simulink model "Heat_Exchanger"  (R2024a)
settings: Solver=FixedStepAuto  StartTime=0.0  StopTime=Inf  RelTol=1e-3
model workspace (MAT data in the model file):
  Avg_HI = 400
  PLC_IP_Address = '127.0.0.1'
libraries: dspnetwork x26
settings Model: Creator=antho  LastModifiedBy=chach
settings SolverCC: AlgebraicLoopSolver=TrustRegion
settings DataIOCC: ReturnWorkspaceOutputs=off
settings OptimizationCC: LifeSpan=inf
settings DebuggingCC: UnconnectedInputMsg=warning  UnconnectedOutputMsg=warning  UnconnectedLineMsg=warning  SFExecutionAtInitializationDiag=none  ArithmeticOperatorsInVariantConditions=warning
settings ModelReferenceCC: EnableRefExpFcnMdlSchedulingChecks=on
settings SFSimCC: SimUseLocalCustomCode=off  CustomCodeUndefinedFunction=UseInterfaceOnly
settings RTWCC: PackageGeneratedCodeAndArtifacts=on  PackageName=Heat_Exchanger  RTWUseLocalCustomCode=off  GPUComputeCapability=3.5
settings CodeAppCC: StateflowObjectComments=on

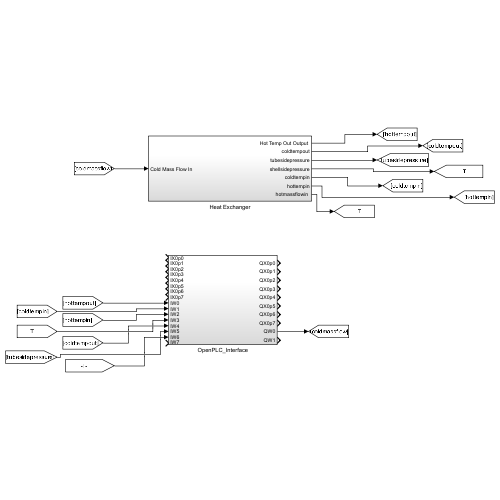
[thumbnail: Simulink's stored preview of the top-level diagram]
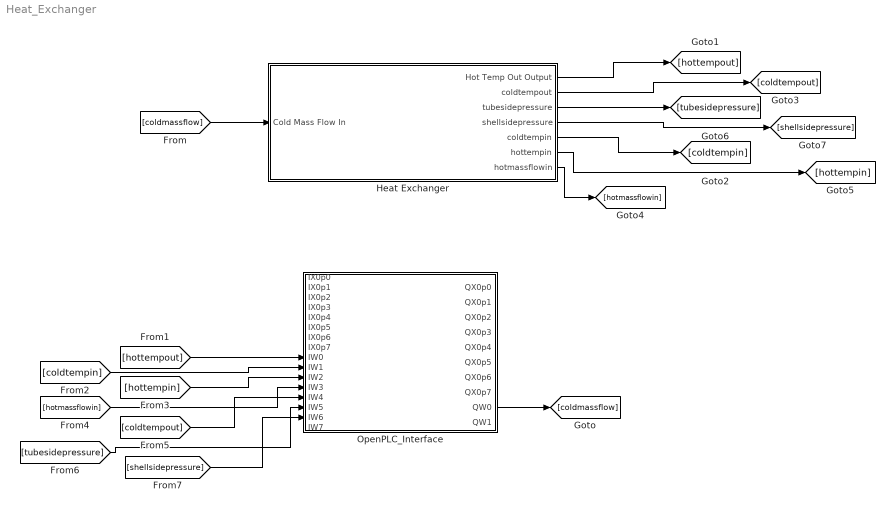
== system Heat_Exchanger ==
  Heat Exchanger : Subsystem
  OpenPLC_Interface : Subsystem
  wires:
  OpenPLC_Interface/9(QW0) -> [coldmassflow]
  [hottempout] -> OpenPLC_Interface/9(IW0)
  [coldtempin] -> OpenPLC_Interface/10(IW1)
  [hottempin] -> OpenPLC_Interface/11(IW2)
  [hotmassflowin] -> OpenPLC_Interface/12(IW3)
  [coldtempout] -> OpenPLC_Interface/13(IW4)
  [tubesidepressure] -> OpenPLC_Interface/14(IW5)
  [shellsidepressure] -> OpenPLC_Interface/15(IW6)
  Heat Exchanger/1("Hot Temp Out Output ") -> [hottempout]
  Heat Exchanger/2(coldtempout) -> [coldtempout]
  Heat Exchanger/3(tubesidepressure) -> [tubesidepressure]
  Heat Exchanger/4(shellsidepressure) -> [shellsidepressure]
  Heat Exchanger/5(coldtempin) -> [coldtempin]
  Heat Exchanger/7("hotmassflowin ") -> [hotmassflowin]
  Heat Exchanger/6(hottempin) -> [hottempin]
  [coldmassflow] -> Heat Exchanger/1(Cold Mass Flow In)

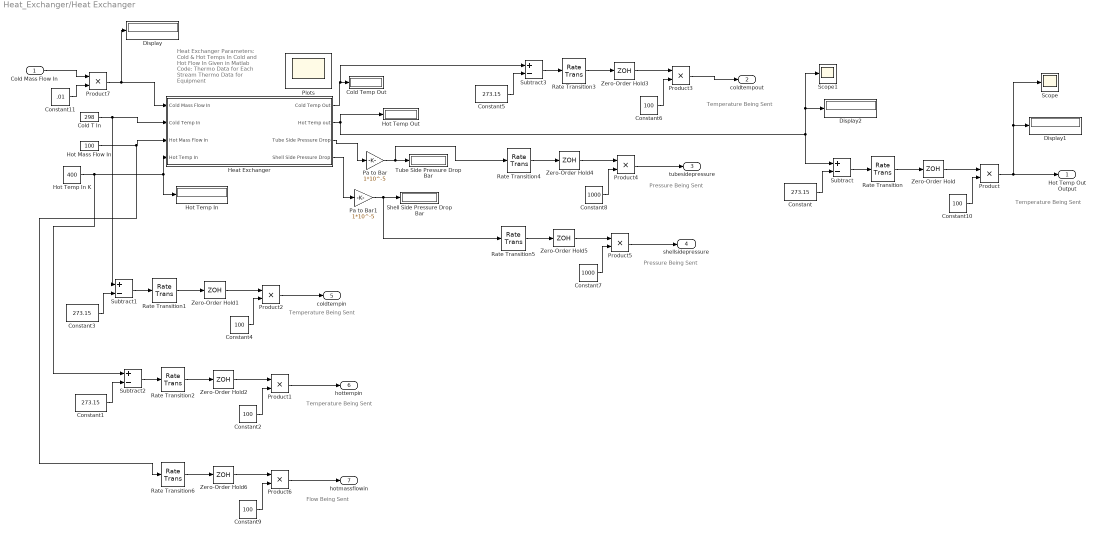
== system Heat_Exchanger/Heat Exchanger ==
  note: Heat Exchanger Parameters:
      | Cold & Hot Temps In
      | Cold and Hot Flow In
      | Given in Matlab Code:
      | Thermo Data for Each Stream
      | Thermo Data for Equipment
  note: Temperature Being Sent
  note: Temperature Being Sent
  note: Temperature Being Sent
  note: Pressure Being Sent
  note: Pressure Being Sent
  note: Flow Being Sent
  note: Temperature Being Sent
  Cold Mass Flow In : Inport
  Cold T In : Constant  Value=298
  Cold Temp Out : Display
  Constant{,1,3,5} (4 alike) : Constant  Value=273.15
  Constant{2,4,6,9..10} (5 alike) : Constant  Value=100
  Constant11 : Constant  Value=.01
  Constant7 : Constant  Value=1000
  Constant8 : Constant  Value=1000
  Display : Display
  Display1 : Display
  Display2 : Display
  Heat Exchanger : Subsystem
  Hot Mass Flow In : Constant  Value=100
  Hot Temp In : Display
  Hot Temp In K : Constant  Value=400
  Hot Temp Out : Display
  Pa to Bar : Gain  Gain=1*10^-5
  Pa to Bar1 : Gain  Gain=1*10^-5
  Plots : Scope
      settings: Floating=on
  Product{,1..7} (8 alike) : Product
  Rate Transition{,1..6} (7 alike) : RateTransition
  Scope : Scope
  Scope1 : Scope
  Shell Side Pressure Drop Bar : Display
  Subtract{,1..3} (4 alike) : Sum  Inputs=+-
  Tube Side Pressure Drop Bar : Display
  Zero-Order Hold{,1..6} (7 alike) : ZeroOrderHold  SampleTime=0.1
  "Hot Temp Out Output " : Outport
  coldtempout : Outport  Port=2
  tubesidepressure : Outport  Port=3
  shellsidepressure : Outport  Port=4
  coldtempin : Outport  Port=5
  hottempin : Outport  Port=6
  "hotmassflowin " : Outport  Port=7
  wires:
  Heat Exchanger/1(Cold Temp Out) -> Subtract3/1, Cold Temp Out/1
  Cold T In/1 -> Subtract1/1, Heat Exchanger/2(Cold Temp In)
  Hot Temp In K/1 -> Subtract2/1, Heat Exchanger/4(Hot Temp In), Hot Temp In/1
  Hot Mass Flow In/1 -> Rate Transition6/1, Heat Exchanger/3(Hot Mass Flow In)
  Pa to Bar/1 -> Rate Transition4/1, Tube Side Pressure Drop Bar/1
  Heat Exchanger/3(Tube Side Pressure Drop) -> Pa to Bar/1
  Pa to Bar1/1 -> Rate Transition5/1, Shell Side Pressure Drop Bar/1
  Heat Exchanger/4(Shell Side Pressure Drop) -> Pa to Bar1/1
  Product2/1 -> coldtempin/1
  Subtract1/1 -> Rate Transition1/1
  Zero-Order Hold1/1 -> Product2/1
  Constant4/1 -> Product2/2
  Constant3/1 -> Subtract1/2
  Rate Transition1/1 -> Zero-Order Hold1/1
  Product1/1 -> hottempin/1
  Subtract2/1 -> Rate Transition2/1
  Zero-Order Hold2/1 -> Product1/1
  Constant2/1 -> Product1/2
  Constant1/1 -> Subtract2/2
  Rate Transition2/1 -> Zero-Order Hold2/1
  Product3/1 -> coldtempout/1
  Subtract3/1 -> Rate Transition3/1
  Zero-Order Hold3/1 -> Product3/1
  Constant6/1 -> Product3/2
  Constant5/1 -> Subtract3/2
  Rate Transition3/1 -> Zero-Order Hold3/1
  Product4/1 -> tubesidepressure/1
  Zero-Order Hold4/1 -> Product4/1
  Constant8/1 -> Product4/2
  Rate Transition4/1 -> Zero-Order Hold4/1
  Zero-Order Hold5/1 -> Product5/1
  Product5/1 -> shellsidepressure/1
  Rate Transition5/1 -> Zero-Order Hold5/1
  Constant7/1 -> Product5/2
  Zero-Order Hold6/1 -> Product6/1
  Product6/1 -> "hotmassflowin "/1
  Rate Transition6/1 -> Zero-Order Hold6/1
  Constant9/1 -> Product6/2
  Subtract/1 -> Rate Transition/1
  Heat Exchanger/2(Hot Temp out) -> Subtract/1, Scope1/1, Display2/1, Hot Temp Out/1
  Constant10/1 -> Product/2
  Constant/1 -> Subtract/2
  Rate Transition/1 -> Zero-Order Hold/1
  Product/1 -> "Hot Temp Out Output "/1, Scope/1, Display1/1
  Zero-Order Hold/1 -> Product/1
  Constant11/1 -> Product7/2
  Cold Mass Flow In/1 -> Product7/1
  Product7/1 -> Display/1, Heat Exchanger/1(Cold Mass Flow In)

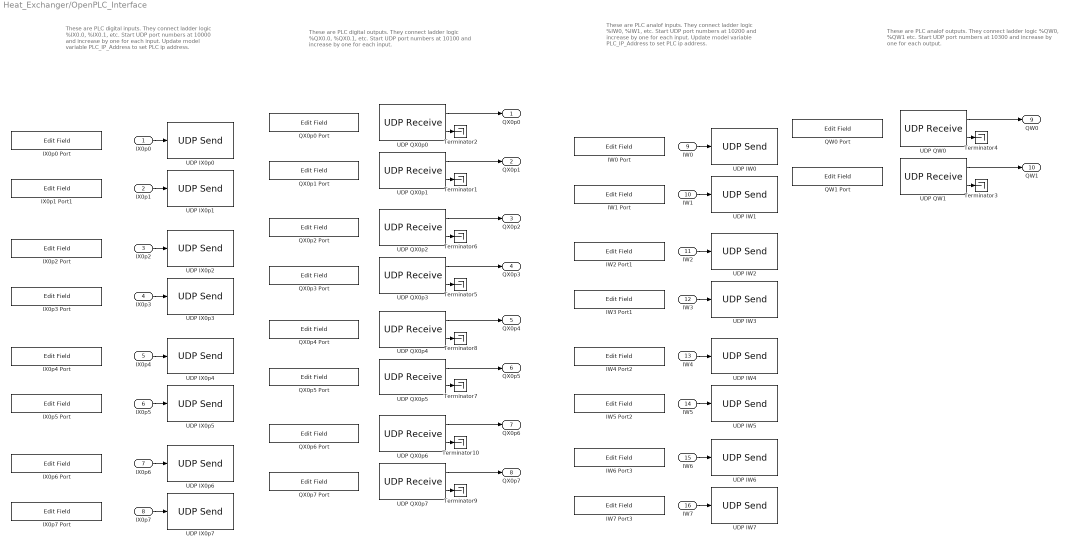
== system Heat_Exchanger/OpenPLC_Interface ==
  note: These are PLC digital inputs. They connect
      | ladder logic %IX0.0, %IX0.1, etc.
      |
      | Start UDP port numbers at 10000 and
      | increase by one for each input.
      |
      | Update model variable PLC_IP_Address
      | to set PLC ip address.
  note: These are PLC digital outputs. They connect
      | ladder logic %QX0.0, %QX0.1, etc.
      |
      | Start UDP port numbers at 10100 and increase
      | by one for each input.
  note: These are PLC analof inputs. They connect
      | ladder logic %IW0, %IW1, etc.
      |
      | Start UDP port numbers  at 10200 and
      | increase by one for each input.
      |
      | Update model variable PLC_IP_Address
      | to set PLC ip address.
  note: These are PLC analof outputs. They connect
      | ladder logic %QW0, %QW1 etc.
      |
      | Start UDP port numbers at 10300 and increase
      | by one for each output.
  "IX0p0 " : Inport
  IX0p1 : Inport  Port=2
  IX0p2 : Inport  Port=3
  IX0p3 : Inport  Port=4
  IX0p4 : Inport  Port=5
  IX0p5 : Inport  Port=6
  IX0p6 : Inport  Port=7
  IX0p7 : Inport  Port=8
  IW0 : Inport  Port=9
  IW1 : Inport  Port=10
  IW2 : Inport  Port=11
  IW3 : Inport  Port=12
  IW4 : Inport  Port=13
  IW5 : Inport  Port=14
  IW6 : Inport  Port=15
  IW7 : Inport  Port=16
  IW0 Port : EditField  LabelPosition=Hide  ShowInitialText=on  Alignment=Center
  IW1 Port : EditField  LabelPosition=Hide  ShowInitialText=on  Alignment=Center
  IW2 Port1 : EditField  LabelPosition=Hide  ShowInitialText=on  Alignment=Center
  IW3 Port1 : EditField  LabelPosition=Hide  ShowInitialText=on  Alignment=Center
  IW4 Port2 : EditField  LabelPosition=Hide  ShowInitialText=on  Alignment=Center
  IW5 Port2 : EditField  LabelPosition=Hide  ShowInitialText=on  Alignment=Center
  IW6 Port3 : EditField  LabelPosition=Hide  ShowInitialText=on  Alignment=Center
  IW7 Port3 : EditField  LabelPosition=Hide  ShowInitialText=on  Alignment=Center
  IX0p0 Port : EditField  LabelPosition=Hide  ShowInitialText=on  Alignment=Center
  IX0p1 Port1 : EditField  LabelPosition=Hide  ShowInitialText=on  Alignment=Center
  IX0p2 Port : EditField  LabelPosition=Hide  ShowInitialText=on  Alignment=Center
  IX0p3 Port : EditField  LabelPosition=Hide  ShowInitialText=on  Alignment=Center
  IX0p4 Port : EditField  LabelPosition=Hide  ShowInitialText=on  Alignment=Center
  IX0p5 Port : EditField  LabelPosition=Hide  ShowInitialText=on  Alignment=Center
  IX0p6 Port : EditField  LabelPosition=Hide  ShowInitialText=on  Alignment=Center
  IX0p7 Port : EditField  LabelPosition=Hide  ShowInitialText=on  Alignment=Center
  QW0 Port : EditField  LabelPosition=Hide  ShowInitialText=on  Alignment=Center
  QW1 Port : EditField  LabelPosition=Hide  ShowInitialText=on  Alignment=Center
  QX0p0 Port : EditField  LabelPosition=Hide  ShowInitialText=on  Alignment=Center
  QX0p1 Port : EditField  LabelPosition=Hide  ShowInitialText=on  Alignment=Center
  QX0p2 Port : EditField  LabelPosition=Hide  ShowInitialText=on  Alignment=Center
  QX0p3 Port : EditField  LabelPosition=Hide  ShowInitialText=on  Alignment=Center
  QX0p4 Port : EditField  LabelPosition=Hide  ShowInitialText=on  Alignment=Center
  QX0p5 Port : EditField  LabelPosition=Hide  ShowInitialText=on  Alignment=Center
  QX0p6 Port : EditField  LabelPosition=Hide  ShowInitialText=on  Alignment=Center
  QX0p7 Port : EditField  LabelPosition=Hide  ShowInitialText=on  Alignment=Center
  Terminator{1..10} (10 alike) : Terminator
  UDP IW0 : dspnetwork/UDP Send  remoteURL='localhost'  remotePort=10200  localURL='255.255.255.255'  localPortSource=Automatically determine  localPort=-1  sendBufferSize=8192  sampletime=-1  blockPlatform=LINUX  separateLengthPort=0
  UDP IW1 : dspnetwork/UDP Send  remoteURL='localhost'  remotePort=10201  localURL='255.255.255.255'  localPortSource=Automatically determine  localPort=-1  sendBufferSize=8192  sampletime=-1  blockPlatform=LINUX  separateLengthPort=0
  UDP IW2 : dspnetwork/UDP Send  remoteURL='localhost'  remotePort=10202  localURL='255.255.255.255'  localPortSource=Automatically determine  localPort=-1  sendBufferSize=8192  sampletime=-1  blockPlatform=LINUX  separateLengthPort=0
  UDP IW3 : dspnetwork/UDP Send  remoteURL='localhost'  remotePort=10203  localURL='255.255.255.255'  localPortSource=Automatically determine  localPort=-1  sendBufferSize=8192  sampletime=-1  blockPlatform=LINUX  separateLengthPort=0
  UDP IW4 : dspnetwork/UDP Send  remoteURL='localhost'  remotePort=10204  localURL='255.255.255.255'  localPortSource=Automatically determine  localPort=-1  sendBufferSize=8192  sampletime=-1  blockPlatform=LINUX  separateLengthPort=0
  UDP IW5 : dspnetwork/UDP Send  remoteURL='localhost'  remotePort=10205  localURL='255.255.255.255'  localPortSource=Automatically determine  localPort=-1  sendBufferSize=8192  sampletime=-1  blockPlatform=LINUX  separateLengthPort=0
  UDP IW6 : dspnetwork/UDP Send  remoteURL='localhost'  remotePort=10206  localURL='255.255.255.255'  localPortSource=Automatically determine  localPort=-1  sendBufferSize=8192  sampletime=-1  blockPlatform=LINUX  separateLengthPort=0
  UDP IW7 : dspnetwork/UDP Send  remoteURL='localhost'  remotePort=10207  localURL='255.255.255.255'  localPortSource=Automatically determine  localPort=-1  sendBufferSize=8192  sampletime=-1  blockPlatform=LINUX  separateLengthPort=0
  UDP IX0p0 : dspnetwork/UDP Send  remoteURL='localhost'  remotePort=10000  localURL='255.255.255.255'  localPortSource=Automatically determine  localPort=-1  sendBufferSize=8192  sampletime=-1  blockPlatform=LINUX  separateLengthPort=0
  UDP IX0p1 : dspnetwork/UDP Send  remoteURL='localhost'  remotePort=10001  localURL='255.255.255.255'  localPortSource=Automatically determine  localPort=-1  sendBufferSize=8192  sampletime=-1  blockPlatform=LINUX  separateLengthPort=0
  UDP IX0p2 : dspnetwork/UDP Send  remoteURL='localhost'  remotePort=10002  localURL='255.255.255.255'  localPortSource=Automatically determine  localPort=-1  sendBufferSize=8192  sampletime=-1  blockPlatform=LINUX  separateLengthPort=0
  UDP IX0p3 : dspnetwork/UDP Send  remoteURL='localhost'  remotePort=10003  localURL='255.255.255.255'  localPortSource=Automatically determine  localPort=-1  sendBufferSize=8192  sampletime=-1  blockPlatform=LINUX  separateLengthPort=0
  UDP IX0p4 : dspnetwork/UDP Send  remoteURL='localhost'  remotePort=10004  localURL='255.255.255.255'  localPortSource=Automatically determine  localPort=-1  sendBufferSize=8192  sampletime=-1  blockPlatform=LINUX  separateLengthPort=0
  UDP IX0p5 : dspnetwork/UDP Send  remoteURL='localhost'  remotePort=10005  localURL='255.255.255.255'  localPortSource=Automatically determine  localPort=-1  sendBufferSize=8192  sampletime=-1  blockPlatform=LINUX  separateLengthPort=0
  UDP IX0p6 : dspnetwork/UDP Send  remoteURL='localhost'  remotePort=10006  localURL='255.255.255.255'  localPortSource=Automatically determine  localPort=-1  sendBufferSize=8192  sampletime=-1  blockPlatform=LINUX  separateLengthPort=0
  UDP IX0p7 : dspnetwork/UDP Send  remoteURL='localhost'  remotePort=10007  localURL='255.255.255.255'  localPortSource=Automatically determine  localPort=-1  sendBufferSize=8192  sampletime=-1  blockPlatform=LINUX  separateLengthPort=0
  UDP QW0 : dspnetwork/UDP Receive  localURL='0.0.0.0'  localPort=10300  remoteURL='0.0.0.0'  remotePort=-1  recvBufferSize=2  dims=1  signalDatatype=uint16  isComplex=off  isVarSize=off  showBlockingTime=on  blockingTime=0  sampletime=0.01  blockPlatform=LINUX
  UDP QW1 : dspnetwork/UDP Receive  localURL='0.0.0.0'  localPort=10301  remoteURL='0.0.0.0'  remotePort=-1  recvBufferSize=2  dims=1  signalDatatype=uint16  isComplex=off  isVarSize=off  showBlockingTime=on  blockingTime=0  sampletime=0.01  blockPlatform=LINUX
  UDP QX0p0 : dspnetwork/UDP Receive  localURL='0.0.0.0'  localPort=10100  remoteURL='0.0.0.0'  remotePort=-1  recvBufferSize=2  dims=1  signalDatatype=uint16  isComplex=off  isVarSize=off  showBlockingTime=on  blockingTime=0  sampletime=0.01  blockPlatform=LINUX
  UDP QX0p1 : dspnetwork/UDP Receive  localURL='0.0.0.0'  localPort=10101  remoteURL='0.0.0.0'  remotePort=-1  recvBufferSize=2  dims=1  signalDatatype=uint16  isComplex=off  isVarSize=off  showBlockingTime=on  blockingTime=0  sampletime=0.01  blockPlatform=LINUX
  UDP QX0p2 : dspnetwork/UDP Receive  localURL='0.0.0.0'  localPort=10102  remoteURL='0.0.0.0'  remotePort=-1  recvBufferSize=2  dims=1  signalDatatype=uint16  isComplex=off  isVarSize=off  showBlockingTime=on  blockingTime=0  sampletime=0.01  blockPlatform=LINUX
  UDP QX0p3 : dspnetwork/UDP Receive  localURL='0.0.0.0'  localPort=10103  remoteURL='0.0.0.0'  remotePort=-1  recvBufferSize=2  dims=1  signalDatatype=uint16  isComplex=off  isVarSize=off  showBlockingTime=on  blockingTime=0  sampletime=0.01  blockPlatform=LINUX
  UDP QX0p4 : dspnetwork/UDP Receive  localURL='0.0.0.0'  localPort=10104  remoteURL='0.0.0.0'  remotePort=-1  recvBufferSize=2  dims=1  signalDatatype=uint16  isComplex=off  isVarSize=off  showBlockingTime=on  blockingTime=0  sampletime=0.01  blockPlatform=LINUX
  UDP QX0p5 : dspnetwork/UDP Receive  localURL='0.0.0.0'  localPort=10105  remoteURL='0.0.0.0'  remotePort=-1  recvBufferSize=2  dims=1  signalDatatype=uint16  isComplex=off  isVarSize=off  showBlockingTime=on  blockingTime=0  sampletime=0.01  blockPlatform=LINUX
  UDP QX0p6 : dspnetwork/UDP Receive  localURL='0.0.0.0'  localPort=10106  remoteURL='0.0.0.0'  remotePort=-1  recvBufferSize=2  dims=1  signalDatatype=uint16  isComplex=off  isVarSize=off  showBlockingTime=on  blockingTime=0  sampletime=0.01  blockPlatform=LINUX
  UDP QX0p7 : dspnetwork/UDP Receive  localURL='0.0.0.0'  localPort=10107  remoteURL='0.0.0.0'  remotePort=-1  recvBufferSize=2  dims=1  signalDatatype=uint16  isComplex=off  isVarSize=off  showBlockingTime=on  blockingTime=0  sampletime=0.01  blockPlatform=LINUX
  QX0p0 : Outport
  QX0p1 : Outport  Port=2
  QX0p2 : Outport  Port=3
  QX0p3 : Outport  Port=4
  QX0p4 : Outport  Port=5
  QX0p5 : Outport  Port=6
  QX0p6 : Outport  Port=7
  QX0p7 : Outport  Port=8
  QW0 : Outport  Port=9
  QW1 : Outport  Port=10
  wires:
  IX0p1/1 -> UDP IX0p1/1
  "IX0p0 "/1 -> UDP IX0p0/1
  UDP QX0p0/1 -> QX0p0/1
  UDP QX0p0/2 -> Terminator2/1
  UDP QX0p1/2 -> Terminator1/1
  UDP QX0p1/1 -> QX0p1/1
  IW1/1 -> UDP IW1/1
  IW0/1 -> UDP IW0/1
  UDP QW1/1 -> QW1/1
  UDP QW1/2 -> Terminator3/1
  UDP QW0/2 -> Terminator4/1
  UDP QW0/1 -> QW0/1
  IX0p2/1 -> UDP IX0p2/1
  IX0p3/1 -> UDP IX0p3/1
  IX0p7/1 -> UDP IX0p7/1
  IX0p6/1 -> UDP IX0p6/1
  IX0p4/1 -> UDP IX0p4/1
  IX0p5/1 -> UDP IX0p5/1
  UDP QX0p2/1 -> QX0p2/1
  UDP QX0p2/2 -> Terminator6/1
  UDP QX0p3/1 -> QX0p3/1
  UDP QX0p3/2 -> Terminator5/1
  UDP QX0p7/2 -> Terminator9/1
  UDP QX0p7/1 -> QX0p7/1
  UDP QX0p6/1 -> QX0p6/1
  UDP QX0p6/2 -> Terminator10/1
  UDP QX0p4/1 -> QX0p4/1
  UDP QX0p4/2 -> Terminator8/1
  UDP QX0p5/1 -> QX0p5/1
  UDP QX0p5/2 -> Terminator7/1
  IW3/1 -> UDP IW3/1
  IW2/1 -> UDP IW2/1
  IW5/1 -> UDP IW5/1
  IW4/1 -> UDP IW4/1
  IW7/1 -> UDP IW7/1
  IW6/1 -> UDP IW6/1

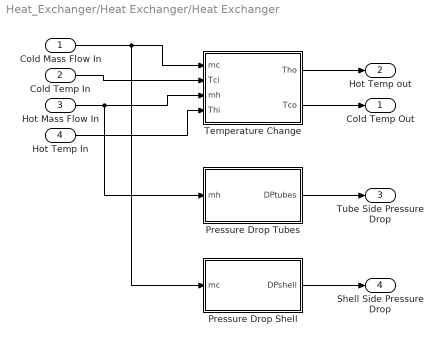
== system Heat_Exchanger/Heat Exchanger/Heat Exchanger ==
  Cold Mass Flow In : Inport
  Cold Temp In : Inport  Port=2
  Hot Mass Flow In : Inport  Port=3
  Hot Temp In : Inport  Port=4
  Pressure Drop Shell : MATLAB Function  TreatAsAtomicUnit=on
  Pressure Drop Tubes : MATLAB Function  TreatAsAtomicUnit=on
  Temperature Change : MATLAB Function  TreatAsAtomicUnit=on
  Cold Temp Out : Outport
  Hot Temp out : Outport  Port=2
  Tube Side Pressure Drop : Outport  Port=3
  Shell Side Pressure Drop : Outport  Port=4
  wires:
  Cold Temp In/1 -> Temperature Change/2(Tci)
  Hot Mass Flow In/1 -> Pressure Drop Tubes/1(mh), Temperature Change/3(mh)
  Cold Mass Flow In/1 -> Pressure Drop Shell/1(mc), Temperature Change/1(mc)
  Temperature Change/2(Tco) -> Cold Temp Out/1
  Pressure Drop Shell/1(DPshell) -> Shell Side Pressure Drop/1
  Temperature Change/1(Tho) -> Hot Temp out/1
  Pressure Drop Tubes/1(DPtubes) -> Tube Side Pressure Drop/1
  Hot Temp In/1 -> Temperature Change/4(Thi)

== matlab function Heat_Exchanger/Heat Exchanger/Heat Exchanger/Pressure Drop Tubes ==
  data: mh input; DPtubes output
function DPtubes = fcn(mh)

densityh=719.15;%kg/m^3
f=0.05;
L=10.9728; %meters
twall=0.0021082;%m
Do=0.028575;%m
Di=(Do-2*twall);
v=((mh/densityh)/24)/(3.14159*(Do-2*twall)^2/4); %Average velocity
DPtubes=f*densityh*v*L/(2*Di);

DPtubes;
end

== matlab function Heat_Exchanger/Heat Exchanger/Heat Exchanger/Temperature Change ==
  data: mc input; Tci input; mh input; Tho output; Thi input; Tco output
function [Tho, Tco]= fcn(mc,Tci,mh,Thi)
    %{
    function Tho = solve(Thi, Tci, Cph, Cpc, mh, mc, A, U) %Generates the output temp of hot stream
       Tho=0;
       n=10*(Thi-Tci)-1;
       for i=0:0.1:n %Iteratively solve for Temperature
           T=Thi-.1*i;
           %Equation to solve for Thi given a "Try Value"
           Tco=((mh*Cph)/(mc*Cpc))*(Thi-T)+Tci;
           DTlm=((T-Tci)-(Thi-Tco))/(log((T-Tci)/(Thi-Tco)));
           Thotry=Thi-((U*A)/(mh*Cph))*DTlm;
           ab=abs(Thotry-T);
           %Checks for solution to problem every iteration
           if 1>ab
               Tho=Thotry;
               break;
           end
       end
        Tho;
    end
    %%%%%%%%%%%%%%%%%%%%%%%%%%%%%%%%%%%%%%%%%%%%%%%%%%%%%%%%%%%%%%%%%%%%%%%%%%%
    function h = calch(v, mu, D, k, density, Cp, ndit)%Generates h given flow rate and heat exchanger parameters
        Re=density*v*D/mu; %Reynolds number
        Pr=Cp*mu/k; %Prandtl number
        h=0.023*Re^0.8*Pr^ndit*k/D; %Dittus-Boelter Correlation
    end
    %}

    %To be input from Simulink%%%%%%%%%%%%%%%%%%%%%%%%%%%%%%%%%%%%%%%%%%%%%%%%%
    %Values shown here might not be equal to those in Simulink. These are here
    %for testing and debugging purposes
    %mc=150;%kg/s
    %mh=100;%kg/s
    %Thi=393;%K
    %Tci=293;%K
    %%%%%%%%%%%%%%%%%%%%%%%%%%%%%%%%%%%%%%%%%%%%%%%%%%%%%%%%%%%%%%%%%%%%%%%%%%%
    %Used for testing and debugging with h functions
    %hh=3305;%W/m^2K
    %hc=6053;%W/m^2K
    %%%%%%%%%%%%%%%%%%%%%%%%%%%%%%%%%%%%%%%%%%%%%%%%%%%%%%%%%%%%%%%%%%%%%%%%%%%

    %General Info on fluids and exchanger%%%%%%%%%%%%%%%%%%%%%%%%%%%%%%%%%%%%%%
    %Cold (c) is Pure Water, Hot (h) is n-octane
    Cpc=4180;%J/kg*K
    Cph=1976;%J/kg*K
    A=400;%m^2
    kw=385;%W/mK
    dxw=0.0021082;%m

    %Calculate h for hot fluid%%%%%%%%%%%%%%%%%%%%%%%%%%%%%%%%%%%%%%%%%%%%%%%%%
    %Tube Side
    muh=0.5195*10^-3;%Pa*s
    Dh=0.028575;%m
    kh=0.137;%W/m*K
    twall=0.0021082;%m
    densityh=719.15;%kg/m^3
    ndith=0.3;%Dittus-Boelter Correlation Power Constant
    ntubes=24;
    vh=((mh/densityh)/ntubes)/(3.14159*(Dh-2*twall)^2/4); %Average velocity
    
    %%CALC H%%
    %hh=calch(vh, muh, Dh, kh, densityh, Cph, ndith);
    Re = densityh*vh*Dh/muh;
    Pr = Cph*muh/kh;
    hh = 0.023*Re^0.8*Pr^ndith*kh/Dh;
    

    %Calculate h for cold fluid%%%%%%%%%%%%%%%%%%%%%%%%%%%%%%%%%%%%%%%%%%%%%%%%
    %Shell Side
    muc=0.6184*10^-3;%Pa*s
    Dc=0.375;%m
    kc=0.107;%W/m*K
    twall=0.0021082;%m
    densityc=919;%kg/m^3
    nditc=0.4;%Dittus-Boelter Correlation Power Constant
    %ntubes=1;
    pt=0.03175; %m
    Dotl=Dh*(ntubes/0.319)^(1/2.142);
    Lb=0.4*Dc;
    Sm=Lb*(Dc-Dotl*((Dotl-Dh)/pt)*(pt-Dh));
    Vc=mc/densityc;
    vc=Vc/Sm;
    
    %%CALC H%%
    %hc=calch(vc, muc, Dc, kc, densityc, Cpc, nditc);
    Re = densityc*vc*Dc/muc;
    Pr = Cpc*muc/kc;
    hc = 0.023*Re^0.8*Pr^nditc*kc/Dc;

    U=1/(1/hh+dxw/kw+1/hc); %Overall Heat Transfer Coefficient

    %solve for the output temperature%%%%%%%%%%%%%%%%%%%%%%%%%
    Tho=0;
    n=10*(Thi-Tci)-1;
    for i=0:0.1:n %Iteratively solve for Temperature
        T=Thi-.1*i;
        %Equation to solve for Thi given a "Try Value"
        Tco=((mh*Cph)/(mc*Cpc))*(Thi-T)+Tci;
        DTlm=((T-Tci)-(Thi-Tco))/(log((T-Tci)/(Thi-Tco)));
        Thotry=Thi-((U*A)/(mh*Cph))*DTlm;
        ab=abs(Thotry-T);
        %Checks for solution to problem every iteration
        if 1>ab
           Tho=Thotry;
           break;
        end
    end
    
    %Calculate Tco
    Tco=Tci+mh*Cph*(Thi-Tho)/(mc*Cpc);
    %Return stream temp out values to Simulink system%%%%%%%%%%%%%%%%%%%%%%%
    if mc==0
       Tco=Tci;
       Tho=Thi;
    end
    Tho;
end

== matlab function Heat_Exchanger/Heat Exchanger/Heat Exchanger/Pressure Drop Shell ==
  data: mc input; DPshell output
function DPshell = fcn(mc)
Dh=0.028575;%m
ntubes=24;
muc=0.6184*10^-3;%Pa*s
Dc=0.375;%m
kc=0.107;%W/m*K
twall=0.0021082;%m
densityc=919;%kg/m^3
nditc=0.4;%Dittus-Boelter Correlation Power Constant
pt=0.03175; %m
Dotl=Dh*(ntubes/0.319)^(1/2.142);
Lb=0.4*Dc;
Sm=Lb*(Dc-Dotl*((Dotl-Dh)/pt)*(pt-Dh));
Vc=mc/densityc;
vc=Vc/Sm;
Rec=densityc*vc*Dc/muc; %Reynolhc number
Ls=10.9728; %meters
Lbb=0.2*Ls; %m, Length between baffles
tb=0.0127; %m
Kf=0.272+2490/Rec+(9270*10^3)/(Rec^2)-(10^10)/(Rec^3);
Dsb=0.00635; %m
Ltb=0.03175; %m
Bc=35;
Thetads=acos(1-2*Bc/100);
Dctl=Dotl-Dh;
Thetactl=2*acos((Dc*(1-2*Bc/100))/Dctl)
Fw=(Thetactl-sin(Thetads))/(2*3.14159);
Stb=(3.14159/4)*(((Dh+Ltb)^2-Dh^2)*ntubes*(1-Fw));
Ssb=Dc*Dsb*(3.14159-0.5*Thetads);
rs=Ssb/(Ssb+Stb);
rl=(Ssb+Stb)/Sm;
p=0.8-0.15*(1+rs);
Rb=2.71828^(-1.33*(1+rs)*rl^p);
Lc=0.35*Dc;
Nc=(Dc-2*Lc)/pt;
Ncw=0.8*Lc/pt;
n=Ls/(Lb+tb);
Dpc=(Nc*Kf)*densityc*vc/2;
DPshell=((n+1)+2*Rb*(1+Ncw/Nc))*Dpc;
if mc==0
    DPshell=0;
end

DPshell;
end
